simulink model "MouvementG"  (R2022b)
settings: Solver=VariableStepAuto  StartTime=0.0  StopTime=10.0  RelTol=1e-3
settings Model: Creator=mathissigier  LastModifiedBy=mathissigier

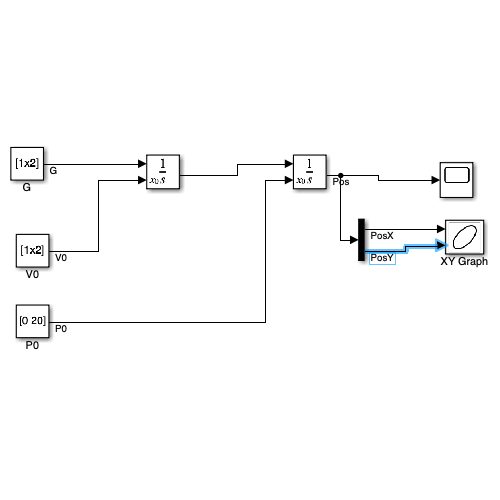
[thumbnail: Simulink's stored preview of the top-level diagram]
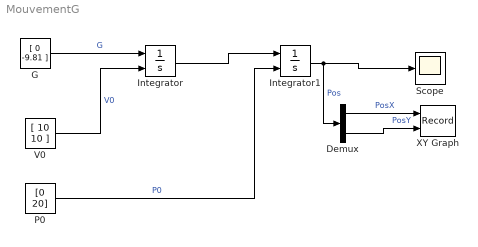
== system MouvementG ==
  Demux : Demux  Outputs=2
  G : Constant  Value=[ 0 -9.81 ]
  Integrator : Integrator  InitialConditionSource=external
  Integrator1 : Integrator  InitialConditionSource=external
  P0 : Constant  Value=[0 20]
  Scope : Scope
  V0 : Constant  Value=[ 10 10 ]
  XY Graph : Record  FileSettingsInternal="{\"entries\":[{\"content\":{\"excelSettings\":{\"content\":{},\"type\":\"Streamout.ExcelSettings\"}},\"type\":\"Streamout.FileSettingStorage\",\"uuid\":\"7a2e6056-7ca3-4c0c-9eb3-d53f51b8aba0\"}],\"packageUris\":[\"http://schema.mathworks.com/mf0/streamout_blocks/R2020a\"],\"version\":\"1.0\"}"  Layout=[1 1]  SignalsInternal="{\"entries\":[{\"content\":{\"signals\":[{\"content\":{\"blockPath\":[\"MouvementG/XY Graph\"],\"channel\":[],\"dimensions\":[1],\"domain\":\"MouvementG/XY Graph\",\"lineColor\":\"#a2142f\",\"plots\":[1],\"port\":1,\"sid\":[\"\"],\"signalID\":74,\"signalName\":\"Demux:1\"},\"type\":\"RecordBlkView.Signal\",\"uuid\":\"17fd00ca-5345-42b9-8e36-00e7819ad670\"},{\"content\":{\"blockPath\":[\"MouvementG/XY Graph\"],\"channel\":[],\"dimensions\":[1],\"domain\":\"MouvementG/XY Graph\",\"lineColor\":\"#139fff\",\"plots\":[1],\"port\":2,\"sid\":[\"\"],\"signalID\":78,\"signalName\":\"Demux:2\"},\"type\":\"RecordBlkView.Signal\",\"uuid\":\"1c44d905-d3e7-4d47-bfa5-47e6144080d4\"}]},\"type\":\"RecordBlkView.InputSignals\",\"uuid\":\"a0698f38-5bee-4173-b1c9-93dd2e082be6\"}],\"packageUris\":[\"http://schema.mathworks.com/mf0/streamout_blocks/R2020a\"],\"version\":\"1.0\"}"  VisualizationBindings="{\"xyplotplugin\":{\"info\":[{\"series\":[{\"bindingParametersList\":[{\"parameter\":\"X-Axis\",\"signalID\":74,\"signalName\":\"Demux:1\"},{\"parameter\":\"Y-Axis\",\"signalID\":78,\"signalName\":\"Demux:2\"}],\"seriesID\":58619}],\"subplotID\":1}]}}"  CompatibilityTag=XY
  wires:
  G/1 -> Integrator/1  "G"
  Integrator/1 -> Integrator1/1
  V0/1 -> Integrator/2  "V0"
  P0/1 -> Integrator1/2  "P0"
  Integrator1/1 -> Demux/1, Scope/1  "Pos"
  Demux/1 -> XY Graph/1  "PosX"
  Demux/2 -> XY Graph/2  "PosY"
